simulink library "Buttons"  (R2018b)
settings: Solver=VariableStepAuto  StartTime=0.0  StopTime=10.0  RelTol=1e-3
settings Model: Creator=rmathijn  LastModifiedBy=Sjoerd

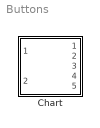
== system Buttons ==
  Chart : Stateflow chart  TreatAsAtomicUnit=on

== stateflow chart Buttons/Chart ==
  state Buttons
    state NoChange
      entry:
      BUTTON_ACTIVITY=false
      exit:
      BUTTON_ACTIVITY=true
    state LSHold
    state RSHold
    state Release
    state ShortPress
    state LongPress
    (default) -> NoChange
    NoChange -> LSHold [order 2] : [leftSensor == 1 && rightSensor == 0]
        | {LHOLD=true}
    NoChange -> RSHold [order 3] : [leftSensor == 0 && rightSensor == 1]
        | {RHOLD=true}
    RSHold -> NoChange : [rightSensor == 0 && leftSensor == 0]
        | {RHOLD=false}
    LSHold -> NoChange : [leftSensor == 0 && rightSensor == 0]
        | {LHOLD=false}
    NoChange -> ShortPress [order 1] : [leftSensor == 1 && rightSensor == 1]
    Release -> NoChange : {SHORT_PRESS=false}
    LongPress -> NoChange : [leftSensor == 0 && rightSensor == 0]
        | {LONG_PRESS=false}
    ShortPress -> Release [order 2] : [leftSensor == 0 && rightSensor == 0]
        | {SHORT_PRESS=true}
    ShortPress -> LongPress [order 1] : [after(1,sec)]{LONG_PRESS=true}
  data: leftSensor input uint8 size=1; rightSensor input uint8 size=1; LHOLD output boolean size=1; RHOLD output boolean size=1; SHORT_PRESS output boolean size=1; LONG_PRESS output boolean size=1; BUTTON_ACTIVITY output boolean size=1
